simulink model "AccTarSel"  (R2018b)
settings: Solver=FixedStepDiscrete  StartTime=0.0  StopTime=inf  FixedStep=0.01  RelTol=1e-3
PostLoadFcn:
  | if any(exist('dsrtsu_mdlpostloadfcn', 'file') ~= 0), dsrtsu_mdlpostloadfcn('Execute', bdroot); end
values from neighbouring files (symbols this model uses):
  P_adtMaxBDC = 1.0    [AccTarSel.sldd]
  P_aFOCApproachIntpAcitve = -0.6    [AccTarSel.sldd]
  P_aFOCApproachIntpEnsure = -1.8    [AccTarSel.sldd]
  P_CutInEnable = 1.0    [AccTarSel.sldd]
  P_dAimMin = 4.5    [AccTarSel.sldd]
  P_dAimMinAVP = 1.5    [AccTarSel.sldd]
  P_dObjDrvOffMax = 5.0    [AccTarSel.sldd]
  P_dObjDrvOffMin = 3.0    [AccTarSel.sldd]
  P_dObjLowHystDecToStop = 4.5    [AccTarSel.sldd]
  P_dObjLowHystDecToStopAVP = 1.5    [AccTarSel.sldd]
  P_dObjUpperHystDecToStop = 5.0    [AccTarSel.sldd]
  P_dResMax = 5.0    [AccTarSel.sldd]
  P_dStandStill = 3.0    [AccTarSel.sldd]
  P_dStandStillMin = 2.0    [AccTarSel.sldd]
  P_dvarYMax4PO = 1.0    [AccTarSel.sldd]
  P_dyCutInThres = 3.6    [AccTarSel.sldd]
  P_facBDCInit = 0.7    [AccTarSel.sldd]
  P_facBDCIterCalc = 0.8    [AccTarSel.sldd]
  P_facFOCNegDiff = 0.3    [AccTarSel.sldd]
  P_facFOCPosDiff = 0.2    [AccTarSel.sldd]
  P_kapHystThres = 0.0005    [AccTarSel.sldd]
  P_PlausIntegDisable = 0.0    [AccTarSel.sldd]
  P_plausMin4PO = 0.5    [AccTarSel.sldd]
  P_probExistMin4PO = 0.8    [AccTarSel.sldd]
  P_StandObjEnable = 0.0    [AccTarSel.sldd]
  P_tAxTrackNegLower = 0.3    [AccTarSel.sldd]
  P_tAxTrackNegUpper = 0.6    [AccTarSel.sldd]
  P_tAxTrackPosLower = 1.0    [AccTarSel.sldd]
  P_tAxTrackPosUpper = 2.0    [AccTarSel.sldd]
  P_tBDCStartFilt = 0.2    [AccTarSel.sldd]
  P_tCSC = 3.5    [AccTarSel.sldd]
  P_tCurvFilt = 0.2    [AccTarSel.sldd]
  P_tCutInFilt = 0.5    [AccTarSel.sldd]
  P_tFiltAxAbsPONegFast = 0.1    [AccTarSel.sldd]
  P_tFiltAxAbsPONegSlow = 0.4    [AccTarSel.sldd]
  P_tFiltAxAbsPOPosFast = 1.2    [AccTarSel.sldd]
  P_tFiltAxAbsPOPosSlow = 2.0    [AccTarSel.sldd]
  P_tFiltAxAbsPOStand = 2.0    [AccTarSel.sldd]
  P_tFiltDAim = 0.1    [AccTarSel.sldd]
  P_tFiltDsd = 0.1    [AccTarSel.sldd]
  P_tFiltSpdLim = 3.0    [AccTarSel.sldd]
  P_tFiltVxAxPOFast = 0.15    [AccTarSel.sldd]
  P_tFiltVxAxPOSlow = 0.25    [AccTarSel.sldd]
  P_tFOCStatAccelFast = 4.0    [AccTarSel.sldd]
  P_tFOCStatAccelSlow = 3.5    [AccTarSel.sldd]
  P_tFOCStatDecelFast = 4.0    [AccTarSel.sldd]
  P_tFOCStatDecelSlow = 3.2    [AccTarSel.sldd]
  P_tMinDrvPhase = 2.0    [AccTarSel.sldd]
  P_tPredObjLeav = 1.2    [AccTarSel.sldd]
  P_tRollingFilt = 0.5    [AccTarSel.sldd]
  P_tRollingFinFilt = 1.0    [AccTarSel.sldd]
  P_tSSCNeg = 4.5    [AccTarSel.sldd]
  P_tSSCPos = 5.5    [AccTarSel.sldd]
  P_tToStop = 5.0    [AccTarSel.sldd]
  P_tToStopInBDC = 6.0    [AccTarSel.sldd]
  P_tToStopTrig = 4.0    [AccTarSel.sldd]
  P_vEgoDecToStop = 3.0    [AccTarSel.sldd]
  P_vEgoLowBDC = 4.0    [AccTarSel.sldd]
  P_vFOCNegDiff = 4.0    [AccTarSel.sldd]
  P_vFOCPosDiff = 5.0    [AccTarSel.sldd]
  P_vFOCStationaryFast = 15.0    [AccTarSel.sldd]
  P_vFOCStationarySlow = 5.0    [AccTarSel.sldd]
  P_vObjDrvOff = 0.5    [AccTarSel.sldd]
  P_vObjLowHystDecToStop = 0.5    [AccTarSel.sldd]
  P_vObjNoStop = 1.0    [AccTarSel.sldd]
  P_vObjReCalc = 1.0    [AccTarSel.sldd]
  P_vObjStop = 0.3    [AccTarSel.sldd]
  P_vObjUpperHystDecToStop = 0.8    [AccTarSel.sldd]
  P_vStandStill = 0.3    [AccTarSel.sldd]
  P_vStandStillHyst = 0.3    [AccTarSel.sldd]
  P_vyCutInThres = 0.5    [AccTarSel.sldd]
libraries: simulink x21, LPFilter x12
(part 1 of 11)
settings Model: DSRTSU_INTERNAL_RTI_VER=540  DSRTSU_INTERNAL_RTI_TYPE=rti1401  RTICANMMDATA=struct('GeneralSetupData',struct('modelroot','C:\Users\linqi\Desktop\matlab\ACC\CarMaker\src_cm4sl','generalsettings',struct('filesettings',struct('destfolder',struct('Name','RTICANMM_FILES','Check',1),'buildfolder',struct('Name','.','Check',1),'AbsDestfolder',struct('Name','C:\Users\linqi\Desktop\matlab\ACC\CarMaker\src_cm4sl\RTICANMM_FILES'),'AbsBuildfolder',struct('Name','C:\Users\linqi\Desktop\matlab\ACC\CarMaker\src_cm4sl'))),'options',struct('addpaths',1,'rmpaths',1,'addtrcexclusion',logical(1),'cannavigator',struct('checkmonitoring',0),'show_usrtrc',0,'use_usrtrc',0),'advanced',struct('options',ones(1,100)),'MPSetup',{{}},'RTI',struct('Type','RTI1401','Ver','7.12','Date','02-May-2019'),'modelname','AccTarSel','block','AccTarSel'))  DSRTSU_INTERNAL_RTIFPGA=130  Creator=linqi  LastModifiedBy=linqi
settings OptimizationCC: BlockReduction=off  ConditionallyExecuteInputs=off  OptimizeBlockIOStorage=off  BufferReuse=off  GlobalBufferReuse=off  ExpressionFolding=off  PassReuseOutputArgsThreshold=0  LocalBlockOutputs=off  OptimizeDataStoreBuffers=off  BusAssignmentInplaceUpdate=off  OptimizationLevel=level0
settings DebuggingCC: ParameterTunabilityLossMsg=error
settings HardwareCC: ProdBitPerPointer=32  ProdBitPerSizeT=32  ProdBitPerPtrDiffT=32  ProdLargestAtomicInteger=Integer  ProdEndianess=BigEndian  ProdWordSize=32  ProdHWDeviceType=Custom Processor->Custom  TargetIntDivRoundTo=Zero  TargetEndianess=BigEndian  TargetHWDeviceType=Custom Processor->Custom
settings ModelReferenceCC: ModelReferenceNumInstancesAllowed=Single
settings SFSimCC: MATLABDynamicMemAlloc=off
settings RTWCC: SystemTargetFile=rti1401.tlc  MakeCommand=make_rti  TemplateMakefile=rti1401.tmf  Description=dSPACE DS1401 Hardware Platform  GenerateReport=on  LaunchReport=on
settings CodeAppCC: OperatorAnnotations=on
settings STFCustomTargetCC: ParMdlRefBuildCompliant=on  SystemTargetFile=rti1401.tlc
settings GRTTargetCC: TargetLangStandard=C89/C90 (ANSI)  CompOptLevelCompliant=off  ConcurrentExecutionCompliant=off  CombineOutputUpdateFcns=off  MatFileLogging=off  CPPClassGenCompliant=off  UseToolchainInfoCompliant=off

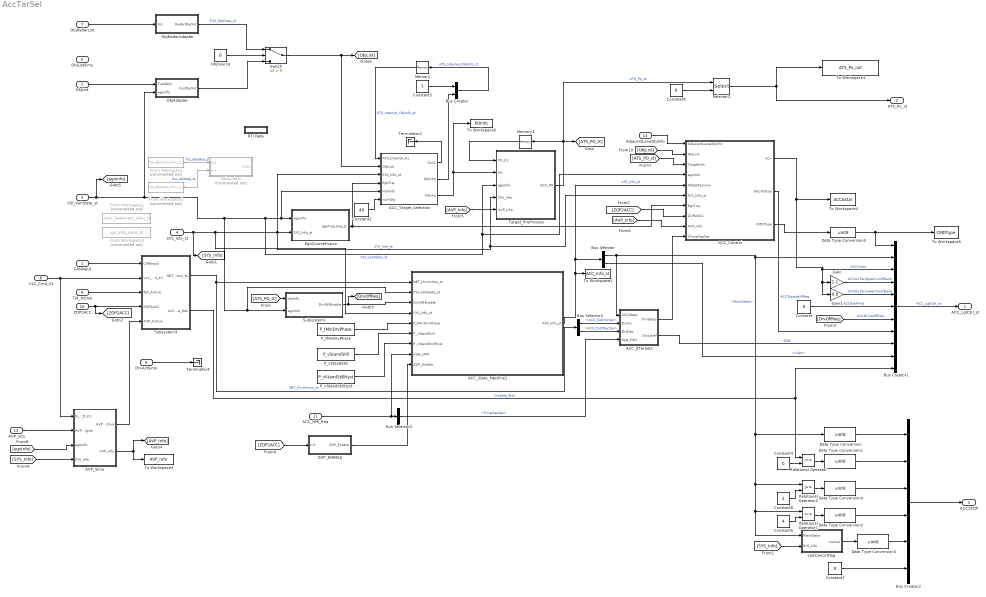
== system AccTarSel ==
  CANInput : Inport  OutDataTypeStr=Bus: COM_VEHBUS_ST  BusOutputAsStruct=on
  ObjList : Inport  Port=2  OutDataTypeStr=Bus: FUS_OBJ_OUTPUT_ST  BusOutputAsStruct=on
  VSI_VehState_st : Inport  Port=3  OutDataTypeStr=Bus: VSI_VEHSTATE_ST  BusOutputAsStruct=on
  SYS_Info_st : Inport  Port=4  OutDataTypeStr=Bus: SYS_INFO_ST  BusOutputAsStruct=on
  ObjListSimu : Inport  Port=5  OutDataTypeStr=Bus: FUS_OBJDATA_ST  BusOutputAsStruct=on
  DrvActSimu : Inport  Port=6  OutDataTypeStr=Bus: NET_DRVACTION_ST  BusOutputAsStruct=on
  ObjRadarList : Inport  Port=7  OutDataTypeStr=Bus: Radar410_Info_ST  BusOutputAsStruct=on
  VLC_Cmd_K1 : Inport  Port=8  OutDataTypeStr=Bus: VLC_LGTCMD_ST  BusOutputAsStruct=on
  TJA_Active : Inport  Port=9
  ZOP2ACC : Inport  Port=10  OutDataTypeStr=Bus: ZOP2ACC  BusOutputAsStruct=on
  ACC_HMI_Req : Inport  Port=11  OutDataTypeStr=Bus: ACC_HMI_REQ
  AVP_Info : Inport  Port=12  OutDataTypeStr=Bus: AVP_OUTPUT_ST  BusOutputAsStruct=on
  AdjacentLaneObjInfo : Inport  Port=13  OutDataTypeStr=Bus: HWA_TARGETOBJECT_OUTPUT_ST  BusOutputAsStruct=on
  ACC_Control : Subsystem
  ACC_State_Machine1 : Stateflow chart  TreatAsAtomicUnit=on
  ACC_Target_Selection : Subsystem  TreatAsAtomicUnit=on
  ACC_dTarSet1 : Subsystem
  AVP_Simu : Subsystem
  Bus Creator : BusCreator  Inputs=2  OutDataTypeStr=Bus: ATS_INTERNAL_OBJINFO_ST  NonVirtualBus=on
  Bus Creator1 : BusCreator  Inputs=11  OutDataTypeStr=Bus: ACC_LGTCTRL_ST  NonVirtualBus=on
      settings: InheritFromInputs=off
  Bus Creator2 : BusCreator  Inputs=6  OutDataTypeStr=Bus: ACC_Status_ST  NonVirtualBus=on
      settings: InheritFromInputs=off
  Bus Selector : BusSelector  OutputSignals=MainState,vSet
  Bus Selector2 : BusSelector  OutputSignals=ACC_DistIncSw,ACC_DistDecSw
  Bus Selector3 : BusSelector  OutputSignals=TimeGapSet
  Constant : Constant  Value=0  OutDataTypeStr=boolean
  Constant2 : Constant  Value=40  OutDataTypeStr=int32
  Constant4 : Constant  Value=0  OutDataTypeStr=uint16
  Constant5 : Constant  OutDataTypeStr=double
  Constant6 : Constant  Value=4  OutDataTypeStr=single
  Constant7 : Constant  Value=0  OutDataTypeStr=uint8
  Constant8 : Constant  Value=2  OutDataTypeStr=single
  Constant9 : Constant  Value=0  OutDataTypeStr=int32
  Data Type Conversion{,1..5} (6 alike) : DataTypeConversion  OutDataTypeStr=uint8
  EgoCourseFusion : Subsystem
  From Workspace : FromWorkspace  Commented=on  VariableName=fus_objdata_simu_1_st  OutDataTypeStr=Bus: FUS_OBJDATA_SIMU_ST  SampleTime=0
  From Workspace1 : FromWorkspace  Commented=on  VariableName=eme_basicinput_simu_st  OutDataTypeStr=Bus: VSI_VEHSTATE_ST  SampleTime=0
  From Workspace2 : FromWorkspace  Commented=on  VariableName=fus_objdata_simu_2_st  OutDataTypeStr=Bus: FUS_OBJDATA_SIMU_ST  SampleTime=0
  From Workspace3 : FromWorkspace  Commented=on  VariableName=sys_info_simu_st  OutDataTypeStr=Bus: SYS_INFO_ST  SampleTime=0
  Gain : Gain  Gain=1.1
  Gain1 : Gain  Gain=0.9
  Memory : Memory
  Memory1 : Memory
  ObjAdapter : Subsystem
  ObjRadarAdapter : Subsystem
  ObjSource : Constant  Value=0  OutDataTypeStr=single
  P_tMinDrvPhase : Constant  Value=P_tMinDrvPhase  OutDataTypeStr=single
  P_vStandStill : Constant  Value=P_vStandStill  OutDataTypeStr=single
  P_vStandStillHyst : Constant  Value=P_vStandStillHyst  OutDataTypeStr=single
  RTI Data : Subsystem  Tag=struct('RTIDataServer',struct('RTIDataServerVs','2','RTIModelDescription','struct(''main'',''AccTarSel'',''sub'',''AccTarSel'',''isMp'',0)'))  LoadFcn="if exist('rtidc'), try,  rtidc('DataHostBlockClbLoad', gcbh); catch, disp(['Warning: ''LoadFcn'' for RTI Data block failed: ' lasterr]); end, end,"  mask(RTI_DATA_HOST){}
      mask help:
      | RTI Data Block.
      | This block is used by RTI to store internal model-dependent data.
      | Please keep this block on the root level of the model. Deleting this block will result in data loss.
      |
      | NEVER DELETE OR COPY THIS BLOCK!
      settings: CopyFcn="if exist('rtidc'), try,  rtidc('DataHostBlockClbCopy', gcbh); catch, disp(['Warning: ''CopyFcn'' for RTI Data block failed: ' lasterr]); end, end,"  DeleteFcn="if exist('rtidc'), try,  rtidc('DataHostBlockClbDelete', gcbh); catch, disp(['Warning: ''DeleteFcn'' for RTI Data block failed: ' lasterr]); end, end,"  ModelCloseFcn="if exist('rtidc'), try,  rtidc('DataHostBlockClbModelClose', gcbh); catch, disp(['Warning: ''ModelCloseFcn'' for RTI Data block failed: ' lasterr]); end, end,"  PreSaveFcn="if exist('rtidc'), try,  rtidc('DataHostBlockClbPreSave', gcbh); catch, disp(['Warning: ''PreSaveFcn'' for RTI Data block failed: ' lasterr]); end, end,"  PostSaveFcn="if exist('rtidc'), try,  rtidc('DataHostBlockClbPostSave', gcbh); catch, disp(['Warning: ''PostSaveFcn'' for RTI Data block failed: ' lasterr]); end, end,"  NameChangeFcn="if exist('rtidc'), try,  rtidc('DataHostBlockClbNameChange', gcbh); catch, disp(['Warning: ''NameChangeFcn'' for RTI Data block failed: ' lasterr]); end, end,"
      mask Help:
      | RTI Data Block.
      | This block is used by RTI to store internal model-dependent data.
      | Please keep this block on the root level of the model. Deleting this block will result in data loss.
      | 
      | NEVER DELETE OR COPY THIS BLOCK!
      mask Display:
      | text(0.5, 0.5, 'RTI Data', 'HorizontalAlignment', 'center');
      | plot([1 0]);
  Relational Operator : RelationalOperator  Operator===  OutDataTypeStr=boolean  RndMeth=Simplest
  Relational Operator1 : RelationalOperator  Operator===  OutDataTypeStr=boolean  RndMeth=Simplest
  Relational Operator2 : RelationalOperator  OutDataTypeStr=boolean  RndMeth=Simplest
  Selector2 : Selector  IndexMode=Zero-based  InputPortWidth=6  IndexOptions=Index vector (port)  Indices=[1 3]  OutputSizes=1
  Subsystem : Subsystem  Commented=on
  Subsystem1 : Subsystem
  Subsystem3 : Subsystem
  Switch : Switch  Criteria=u2 > Threshold
  Target_PreProcess : Subsystem
  Terminator2 : Terminator
  Terminator4 : Terminator
  To Workspace1 : ToWorkspace  VariableName=ATS_Po_out  SaveFormat=Timeseries  SampleTime=-1
  To Workspace2 : ToWorkspace  VariableName=ACC_Info_st  SaveFormat=Timeseries  SampleTime=-1
  To Workspace3 : ToWorkspace  VariableName=AVP_Info  SaveFormat=Timeseries  SampleTime=-1
  To Workspace4 : ToWorkspace  VariableName=ACCAxtar  SaveFormat=Timeseries  SampleTime=-1
  To Workspace5 : ToWorkspace  VariableName=CMDType  SaveFormat=Timeseries  SampleTime=-1
  To Workspace6 : ToWorkspace  VariableName=POInfo  SaveFormat=Timeseries  SampleTime=-1
  ZOP_ENABLE : Subsystem
  calcCancelFlag : Subsystem
  ACC_LgtCtrl_st : Outport  OutDataTypeStr=Bus: ACC_LGTCTRL_ST  BusOutputAsStruct=on
  ATS_Po_st : Outport  Port=2  OutDataTypeStr=Bus: ATS_PO_ST  BusOutputAsStruct=on
  ACC2ZOP : Outport  Port=3  OutDataTypeStr=Bus: ACC_Status_ST  BusOutputAsStruct=on
  wires:
  EgoCourseFusion/1(egoTrajLane_st) -> ACC_Control/7(EgoTraj), ACC_Target_Selection/4(EgoTraj)
  ACC_Target_Selection/1(Out1) -> Terminator2/1
  Bus Creator/1 -> Memory/1  "ATS_Internal_ObjInfo_st"
  Constant5/1 -> Bus Creator/1
  ACC_Target_Selection/2(ObjInfo) -> Bus Creator/2
  Target_PreProcess/1(ACC_PO) -> [ATS_PO_st], Selector2/1, Memory1/1  "ATS_Po_st"
  ACC_State_Machine1/1(AST_Info_st) -> To Workspace2/1, Bus Selector/1, ACC_Control/5(StateMachine)  "AST_Info_st"
  VSI_VehState_st/1 -> [egoInfo], ObjAdapter/2(egoInfo), ACC_State_Machine1/2(VSI_VehState_st), Subsystem1/2(egoInfo), ACC_Control/4(egoInfo), Target_PreProcess/3(egoInfo), EgoCourseFusion/1(egoInfo), ACC_Target_Selection/5(VehInfo)  "VSI_VehState_st"
  ACC_Control/1(aCv) -> Bus Creator1/3, Gain1/1, Gain/1, To Workspace4/1  "ACCAxtar"
  From Workspace/1 -> Subsystem/1(In1)  "fus_objdata_st"
  From Workspace2/1 -> Subsystem/2(In2)  "fus_objdata_st"
  ACC_Control/2("DecToStop ") -> Bus Creator1/8  "ACCStandstillReq"
  [ATS_PO_st] -> Subsystem1/1(objInfo)
  Subsystem1/1(DrvOffEnable) -> ACC_State_Machine1/3(DrvOffEnable), [DrvOffReq]
  P_tMinDrvPhase/1 -> ACC_State_Machine1/5(P_tMinDrvPhase)
  P_vStandStill/1 -> ACC_State_Machine1/6(P_vStandStill)
  Gain/1 -> Bus Creator1/4  "ACCAxTarUpperComfBand"
  Gain1/1 -> Bus Creator1/5  "ACCAxTarLowerComfBand"
  Constant/1 -> Bus Creator1/6  "ACCBrkPrfrd"
  [DrvOffReq] -> Bus Creator1/7  "ACCDriveoffReq"
  Bus Creator1/1 -> ACC_LgtCtrl_st/1  "ACC_LgtCtrl_st"
  SYS_Info_st/1 -> [SYS_Info], ACC_State_Machine1/4(SYS_Info_st), EgoCourseFusion/2(SYS_Info_st), Target_PreProcess/4(SYS_Info), ACC_Control/6(SYS_Info_st), ACC_Target_Selection/3(SYS_Info_st)  "SYS_Info_st"
  Memory/1 -> ACC_Target_Selection/1(ATS_Internal_K1)  "ATS_Internal_ObjInfo_st"
  ObjList/1 -> ObjAdapter/1(FusObjIn)
  CANInput/1 -> Subsystem3/1(CANInput)
  Subsystem3/1(NET_DrvAction_st) -> ACC_State_Machine1/1(NET_DrvAction_st), Bus Selector2/1  "NET_DrvAction_st"
  DrvActSimu/1 -> Terminator4/1
  Bus Selector/2 -> Bus Creator1/10  "<vSet>"
  ObjRadarList/1 -> ObjRadarAdapter/1(In1)
  Constant2/1 -> ACC_Target_Selection/6(numObj)
  ACC_Target_Selection/3(POInfo) -> Target_PreProcess/2(PO), To Workspace6/1
  Memory1/1 -> Target_PreProcess/1(PO_K1)
  P_vStandStillHyst/1 -> ACC_State_Machine1/7(P_vStandStillHyst)
  ObjSource/1 -> Switch/2
  Switch/1 -> [ObjList], ACC_Target_Selection/2(ObjList)
  ObjRadarAdapter/1(RadarObjOut) -> Switch/1  "FUS_ObjData_st"
  ObjAdapter/1(FusObjOut) -> Switch/3
  VLC_Cmd_K1/1 -> AVP_Simu/1("VLC_CMD_K1 "), Subsystem3/2(VLC_Cmd_K1)
  Bus Selector2/1 -> ACC_dTarSet1/2(DisInc)  "<ACC_DistIncSw>"
  Bus Selector2/2 -> ACC_dTarSet1/3(DisDec)  "<ACC_DistDecSw>"
  ACC_dTarSet1/1(TimeGap) -> ACC_Control/10(tTimeGapSet)
  ACC_dTarSet1/2(DisLevel) -> Bus Creator1/9  "dSet"
  Subsystem3/2(ACC_Disable_Msk) -> Bus Creator1/11, Relational Operator/1  "Disable_Msk"
  TJA_Active/1 -> Subsystem3/3(TJA_Active)
  Bus Creator2/1 -> ACC2ZOP/1
  Constant4/1 -> Relational Operator/2
  Data Type Conversion/1 -> Bus Creator2/1
  Relational Operator/1 -> Data Type Conversion1/1
  Data Type Conversion1/1 -> Bus Creator2/2
  Constant6/1 -> Relational Operator1/2
  Relational Operator1/1 -> Data Type Conversion2/1
  Data Type Conversion2/1 -> Bus Creator2/4
  [SYS_Info] -> calcCancelFlag/2(SYS_Info)
  calcCancelFlag/1(Cancel) -> Data Type Conversion3/1
  Data Type Conversion3/1 -> Bus Creator2/5
  Constant7/1 -> Bus Creator2/6
  Relational Operator2/1 -> Data Type Conversion4/1
  Constant8/1 -> Relational Operator2/2
  Bus Selector/1 -> ACC_dTarSet1/1(ACCState), Bus Creator1/2, Relational Operator2/1, calcCancelFlag/1(MainState), Relational Operator1/1, Data Type Conversion/1  "<MainState>"
  Data Type Conversion4/1 -> Bus Creator2/3
  ZOP2ACC/1 -> Subsystem3/4(ZOP2ACC), [ZOP2ACC]
  [ZOP2ACC] -> ACC_Control/8(ZOP2ACC)
  Constant9/1 -> Selector2/2
  Selector2/1 -> ATS_Po_st/1, To Workspace1/1
  Bus Selector3/1 -> ACC_dTarSet1/4(tSet_HMI)  "<TimeGapSet>"
  ACC_HMI_Req/1 -> ACC_State_Machine1/8(vSet_HMI), Bus Selector3/1
  ACC_Control/3(CMDType) -> Data Type Conversion5/1
  Data Type Conversion5/1 -> To Workspace5/1, Bus Creator1/1
  [ZOP2ACC] -> ZOP_ENABLE/1(In1)
  ZOP_ENABLE/1(ZOP_Enable) -> ACC_State_Machine1/9(ZOP_Enable)
  [AVP_Info] -> Target_PreProcess/5(AVP_Info)
  [ATS_PO_st] -> ACC_Control/3(TargetInfo)
  [AVP_Info] -> ACC_Control/9(AVP_Info)
  AVP_Simu/2(AVP_Info) -> [AVP_Info], To Workspace3/1
  AVP_Info/1 -> AVP_Simu/2(AVP_Signal)
  [egoInfo] -> AVP_Simu/3(egoInfo)
  [SYS_Info] -> AVP_Simu/4(SYS_Info)
  AVP_Simu/1(AVP_Active) -> Subsystem3/5(AVP_Active)
  AdjacentLaneObjInfo/1 -> ACC_Control/1(AdjacentLaneObjInfo)
  [ObjList] -> ACC_Control/2(ObjList)

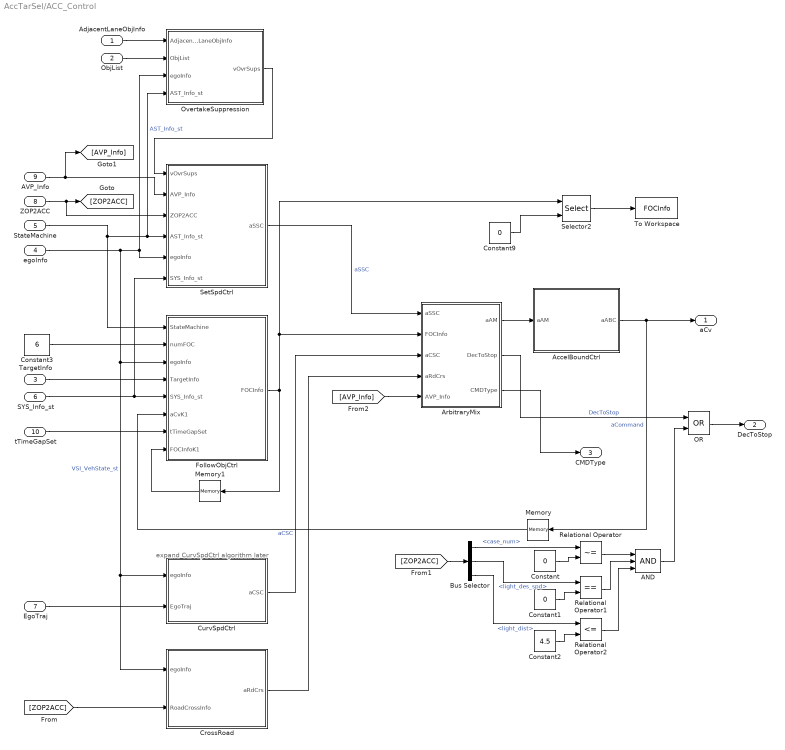
== system AccTarSel/ACC_Control ==
  note: expand CurvSpdCtrl algorithm later
  AdjacentLaneObjInfo : Inport
  ObjList : Inport  Port=2
  TargetInfo : Inport  Port=3
  egoInfo : Inport  Port=4
  StateMachine : Inport  Port=5
  SYS_Info_st : Inport  Port=6
  EgoTraj : Inport  Port=7
  ZOP2ACC : Inport  Port=8
  AVP_Info : Inport  Port=9
  tTimeGapSet : Inport  Port=10
  AND : Logic  Inputs=3  AllPortsSameDT=off  OutDataTypeStr=boolean
  AccelBoundCtrl : Subsystem
  ArbitraryMix : Subsystem
  Bus Selector : BusSelector  OutputSignals=case_num,light_des_spd,light_dist
  Constant : Constant  Value=0  OutDataTypeStr=int8
  Constant1 : Constant  Value=0  OutDataTypeStr=int8
  Constant2 : Constant  Value=4.5  OutDataTypeStr=int8
  Constant3 : Constant  Value=6  OutDataTypeStr=int32
  Constant9 : Constant  Value=0  OutDataTypeStr=int32
  CrossRoad : Subsystem
  CurvSpdCtrl : Subsystem
  FollowObjCtrl : Subsystem
  Memory : Memory
  Memory1 : Memory
  OR : Logic  Operator=OR  AllPortsSameDT=off  OutDataTypeStr=boolean
  OvertakeSuppression : Subsystem
  Relational Operator : RelationalOperator  Operator=~=  OutDataTypeStr=boolean  RndMeth=Simplest
  Relational Operator1 : RelationalOperator  Operator===  OutDataTypeStr=boolean  RndMeth=Simplest
  Relational Operator2 : RelationalOperator  Operator=<=  OutDataTypeStr=boolean  RndMeth=Simplest
  Selector2 : Selector  IndexMode=Zero-based  InputPortWidth=6  IndexOptions=Index vector (port)  Indices=[1 3]  OutputSizes=1
  SetSpdCtrl : Subsystem
  To Workspace : ToWorkspace  VariableName=FOCInfo  SaveFormat=Timeseries  SampleTime=-1
  aCv : Outport
  "DecToStop " : Outport  Port=2
  CMDType : Outport  Port=3
  wires:
  StateMachine/1 -> FollowObjCtrl/1(StateMachine), OvertakeSuppression/4(AST_Info_st), SetSpdCtrl/4(AST_Info_st)  "AST_Info_st"
  egoInfo/1 -> CrossRoad/1(egoInfo), CurvSpdCtrl/1(egoInfo), FollowObjCtrl/3(egoInfo), SetSpdCtrl/5(egoInfo), OvertakeSuppression/3(egoInfo)  "VSI_VehState_st"
  SetSpdCtrl/1(aSSC) -> ArbitraryMix/1(aSSC)  "aSSC"
  TargetInfo/1 -> FollowObjCtrl/4(TargetInfo)
  CurvSpdCtrl/1(aCSC) -> ArbitraryMix/3(aCSC)  "aCSC"
  ArbitraryMix/1(aAM) -> AccelBoundCtrl/1(aAM)
  AccelBoundCtrl/1(aABC) -> aCv/1, Memory/1  "aCommand"
  SYS_Info_st/1 -> SetSpdCtrl/6(SYS_Info_st), FollowObjCtrl/5(SYS_Info_st)
  Memory/1 -> FollowObjCtrl/6(aCvK1)
  tTimeGapSet/1 -> FollowObjCtrl/7(tTimeGapSet)
  EgoTraj/1 -> CurvSpdCtrl/2(EgoTraj)
  ZOP2ACC/1 -> SetSpdCtrl/3(ZOP2ACC), [ZOP2ACC]
  [ZOP2ACC] -> CrossRoad/2(RoadCrossInfo)
  CrossRoad/1(aRdCrs) -> ArbitraryMix/4(aRdCrs)
  [ZOP2ACC] -> Bus Selector/1
  Bus Selector/1 -> Relational Operator/1  "<case_num>"
  Constant/1 -> Relational Operator/2
  Bus Selector/2 -> Relational Operator1/1  "<light_des_spd>"
  Constant1/1 -> Relational Operator1/2
  Bus Selector/3 -> Relational Operator2/1  "<light_dist>"
  Constant2/1 -> Relational Operator2/2
  Relational Operator/1 -> AND/1
  Relational Operator2/1 -> AND/3
  Relational Operator1/1 -> AND/2
  ArbitraryMix/2(DecToStop) -> OR/1  "DecToStop"
  AND/1 -> OR/2
  OR/1 -> "DecToStop "/1
  FollowObjCtrl/1(FOCInfo) -> Selector2/1, ArbitraryMix/2(FOCInfo), Memory1/1
  Memory1/1 -> FollowObjCtrl/8(FOCInfoK1)
  Constant3/1 -> FollowObjCtrl/2(numFOC)
  Constant9/1 -> Selector2/2
  Selector2/1 -> To Workspace/1
  ArbitraryMix/3(CMDType) -> CMDType/1
  AVP_Info/1 -> [AVP_Info], SetSpdCtrl/2(AVP_Info)
  [AVP_Info] -> ArbitraryMix/5(AVP_Info)
  AdjacentLaneObjInfo/1 -> OvertakeSuppression/1(AdjacentLaneObjInfo)
  ObjList/1 -> OvertakeSuppression/2(ObjList)
  OvertakeSuppression/1(vOvrSups) -> SetSpdCtrl/1(vOvrSups)

== system AccTarSel/ACC_Target_Selection ==
  ATS_Internal_K1 : Inport
  ObjList : Inport  Port=2
  SYS_Info_st : Inport  Port=3
  EgoTraj : Inport  Port=4
  VehInfo : Inport  Port=5
  numObj : Inport  Port=6
  Assignment : Assignment  IndexMode=Zero-based  DiagnosticForDimensions=Warning  IndexOptions=Index vector (port)  Indices=1  OutputSizes=1
  Assignment1 : Assignment  IndexMode=Zero-based  DiagnosticForDimensions=Warning  IndexOptions=Index vector (port)  Indices=1  OutputSizes=1
  Bus Selector : BusSelector  OutputSignals=signal2
  Bus Selector1 : BusSelector  OutputSignals=objdata_st
  For Iterator : ForIterator  IterationSource=external  IterationLimit=2  IndexMode=Zero-based
  Selector : Selector  IndexMode=Zero-based  InputPortWidth=40  IndexOptions=Index vector (port)  Indices=[1 3]  OutputSizes=1
  Selector1 : Selector  IndexMode=Zero-based  InputPortWidth=40  IndexOptions=Index vector (port)  Indices=[1 3]  OutputSizes=1
  Subsystem : Subsystem
  TargetSel : Subsystem
  Zero : Constant  Value=zeros(1,40)  OutDataTypeStr=boolean
  Zero1 : Constant  Value=zeros(1,40)  OutDataTypeStr=Bus: ATS_OBJINFO_ST
  Out1 : Outport
  ObjInfo : Outport  Port=2  OutDataTypeStr=Bus: ATS_OBJINFO_ST
  POInfo : Outport  Port=3  OutDataTypeStr=Bus: ATS_PO_ST
  wires:
  For Iterator/1 -> Selector1/2, Assignment1/3, Selector/2, Assignment/3, TargetSel/3(index)  "i_cnt"
  ObjList/1 -> Bus Selector1/1  "fus_objdata_st"
  Bus Selector1/1 -> Selector/1  "<objdata_st>"
  Selector/1 -> Subsystem/1(objInfo), TargetSel/2(objInfo)
  Zero/1 -> Assignment/1
  Assignment/1 -> Out1/1
  Zero1/1 -> Assignment1/1
  Assignment1/1 -> ObjInfo/1
  Subsystem/1(isTargetValid) -> Assignment/2, TargetSel/1(isTargetValid)
  EgoTraj/1 -> Subsystem/2(egoTrajLane_st)  "egoTrajLane_st"
  VehInfo/1 -> [egoInfo], Subsystem/3(VSI_VehState_st)  "VSI_VehState_st"
  Subsystem/2("ats_objInfo ") -> Assignment1/2
  Selector1/1 -> Subsystem/4(ATS_Internal_K1)
  ATS_Internal_K1/1 -> Bus Selector/1
  Bus Selector/1 -> Selector1/1  "<signal2>"
  SYS_Info_st/1 -> Subsystem/5(SYS_Info_st)
  numObj/1 -> For Iterator/1
  TargetSel/1(Out1) -> POInfo/1
  [egoInfo] -> TargetSel/4(egoInfo)

== system AccTarSel/ACC_dTarSet1 ==
  ACCState : Inport
  DisInc : Inport  Port=2
  DisDec : Inport  Port=3
  tSet_HMI : Inport  Port=4
  1-D Lookup Table : Lookup_n-D  NumberOfTableDimensions=1  BreakpointsForDimension1=[1 2 3]  Table=[1.4 1.8 2.1]  InterpMethod=Flat  InternalRulePriority=Speed  RndMeth=Simplest  InputSameDT=on
  AND : Logic  AllPortsSameDT=off  OutDataTypeStr=boolean
  AND1 : Logic  AllPortsSameDT=off  OutDataTypeStr=boolean
  AND2 : Logic  AllPortsSameDT=off  OutDataTypeStr=boolean
  Demux : Demux  Outputs=2
  Equal : RelationalOperator  Operator=~=  OutDataTypeStr=boolean  RndMeth=Simplest
  If Action Subsystem : Subsystem  TreatAsAtomicUnit=on
  If Action Subsystem1 : Subsystem  TreatAsAtomicUnit=on
  If Action Subsystem2 : Subsystem  TreatAsAtomicUnit=on
  If1 : If  NumInputs=2  IfExpression=u1 == 1  ElseIfExpressions=u2 == 1
  Memory : Memory
  Memory1 : Memory  InitialCondition=3
  Merge : Merge  Inputs=3  InitialOutput=0
  Mux : Mux  Inputs=2
  Subsystem : Subsystem
  Switch : Switch  Criteria=u2 > Threshold
  TimeGap : Outport
  DisLevel : Outport  Port=2
  wires:
  If1/1 -> If Action Subsystem/Action
  If Action Subsystem/1(Out1) -> Merge/1
  Memory1/1 -> If Action Subsystem/1(In1), If Action Subsystem1/1(In1), If Action Subsystem2/1(In1)
  If Action Subsystem1/1(Out1) -> Merge/2
  If1/2 -> If Action Subsystem1/Action
  If Action Subsystem2/1(Out1) -> Merge/3
  If1/3 -> If Action Subsystem2/Action
  Subsystem/1(PreCon) -> AND2/2, AND1/1
  AND1/1 -> Memory/1, Equal/1, AND/1
  Memory/1 -> Equal/2
  Equal/1 -> AND/2
  AND/1 -> Demux/1
  Demux/1 -> If1/1
  Demux/2 -> If1/2
  Mux/1 -> AND1/2
  ACCState/1 -> Subsystem/1(ACCState)
  DisInc/1 -> Mux/1
  DisDec/1 -> Mux/2
  1-D Lookup Table/1 -> TimeGap/1
  Switch/1 -> DisLevel/1, Memory1/1, 1-D Lookup Table/1
  Merge/1 -> Switch/3
  tSet_HMI/1 -> AND2/1
  AND2/1 -> Switch/1, Switch/2

== system AccTarSel/AVP_Simu ==
  "VLC_CMD_K1 " : Inport
  AVP_Signal : Inport  Port=2
  egoInfo : Inport  Port=3
  SYS_Info : Inport  Port=4
  AVP_Activate : Subsystem  TreatAsAtomicUnit=on
  AVP_Deactivate : Subsystem  TreatAsAtomicUnit=on
  Bus Selector1 : BusSelector  OutputSignals=ACCState
  Bus Selector8 : BusSelector  OutputSignals=AVP_STATE
  Constant : Constant  OutDataTypeStr=single
  Hold : Subsystem  TreatAsAtomicUnit=on
  If : If  NumInputs=2  IfExpression=u1 == 1  ElseIfExpressions=u2 == 1
  Memory : Memory
  Memory3 : Memory
  Merge : Merge  Inputs=3
  Relational Operator : RelationalOperator  Operator=<=  OutDataTypeStr=boolean  RndMeth=Simplest
  Relational Operator1 : RelationalOperator  Operator=~=  OutDataTypeStr=boolean  RndMeth=Simplest
  Switch : Switch  Criteria=u2 > Threshold
  calcAVPInfo : Subsystem
  default : Subsystem
  AVP_Active : Outport
  AVP_Info : Outport  Port=2
  wires:
  "VLC_CMD_K1 "/1 -> Bus Selector1/1
  egoInfo/1 -> calcAVPInfo/2(egoInfo)
  SYS_Info/1 -> calcAVPInfo/3(SYS_Info)
  Bus Selector1/1 -> Relational Operator/1  "<ACCState>"
  Constant/1 -> Relational Operator/2
  If/1 -> AVP_Activate/Action
  Relational Operator/1 -> If/2
  If/2 -> AVP_Deactivate/Action
  AVP_Activate/1(Out1) -> Merge/1
  AVP_Deactivate/1(Out1) -> Merge/2
  Merge/1 -> [AVP_Active], AVP_Active/1, Memory/1
  Memory/1 -> Hold/1(AVP_ActiveK1)
  If/3 -> Hold/Action
  Hold/1(Out1) -> Merge/3
  Memory3/1 -> Relational Operator1/2
  Relational Operator1/1 -> If/1
  AVP_Signal/1 -> calcAVPInfo/1(AVP_Info), Bus Selector8/1
  Bus Selector8/1 -> Memory3/1, Relational Operator1/1  "<AVP_STATE>"
  [AVP_Active] -> Switch/2
  calcAVPInfo/1(Out1) -> Switch/1
  default/1(Out1) -> Switch/3
  Switch/1 -> AVP_Info/1
